simulink model "second_1"  (R2021b)
settings: Solver=VariableStepAuto  StartTime=0.0  StopTime=10.0  RelTol=1e-3
settings Model: Creator=fredric  LastModifiedBy=fredric

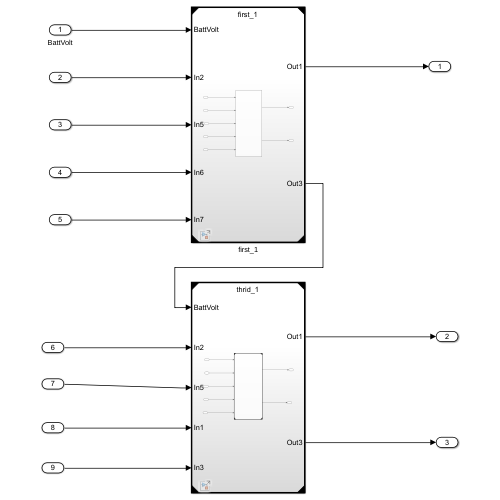
[thumbnail: Simulink's stored preview of the top-level diagram]
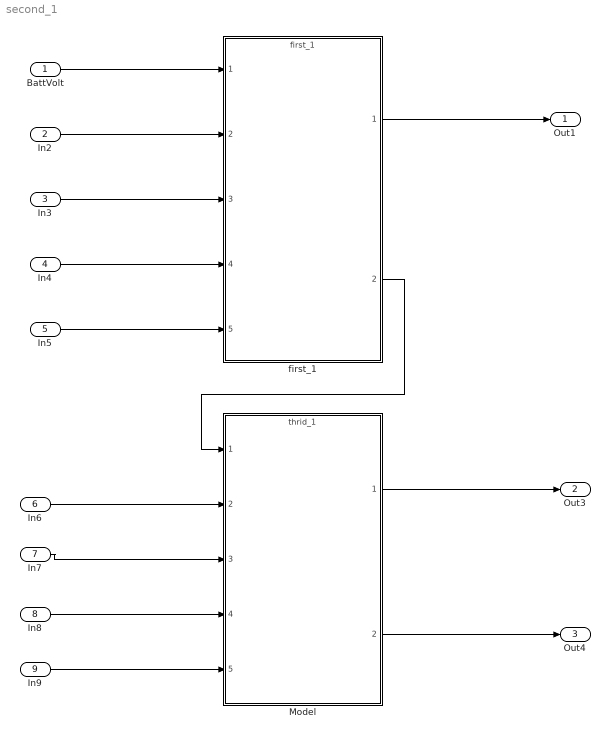
== system second_1 ==
  BattVolt : Inport
  In2 : Inport  Port=2
  In3 : Inport  Port=3
  In4 : Inport  Port=4
  In5 : Inport  Port=5
  In6 : Inport  Port=6
  In7 : Inport  Port=7
  In8 : Inport  Port=8
  In9 : Inport  Port=9
  Model : ModelReference  ModelNameDialog=thrid_1.slx  ModelReferenceVersion=1.8
  first_1 : ModelReference  ModelNameDialog=first_1  ModelReferenceVersion=1.3
  Out1 : Outport
  Out3 : Outport  Port=2
  Out4 : Outport  Port=3
  wires:
  BattVolt/1 -> first_1/1
  In2/1 -> first_1/2
  In3/1 -> first_1/3
  In4/1 -> first_1/4
  In5/1 -> first_1/5
  first_1/1 -> Out1/1
  In6/1 -> Model/2
  In9/1 -> Model/5
  In7/1 -> Model/3
  In8/1 -> Model/4
  Model/1 -> Out3/1
  Model/2 -> Out4/1
  first_1/2 -> Model/1
